simulink model "trajectory_test"  (R2021b)
settings: Solver=VariableStepAuto  StartTime=0.0  StopTime=65  RelTol=1e-3
settings Model: Creator=brian  LastModifiedBy=brian

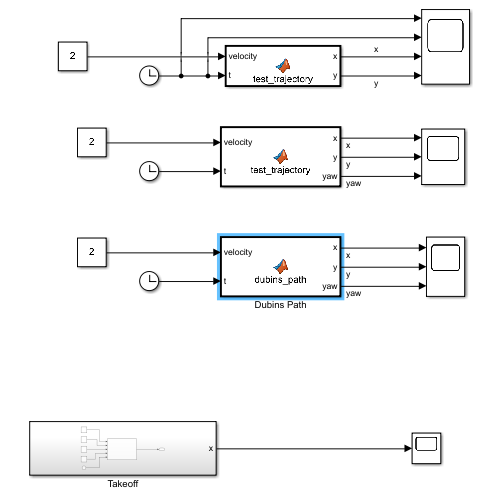
[thumbnail: Simulink's stored preview of the top-level diagram]
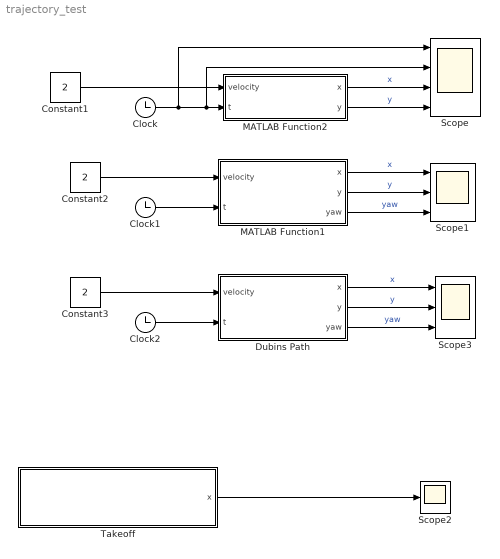
== system trajectory_test ==
  Clock : Clock
  Clock1 : Clock
  Clock2 : Clock
  Constant1 : Constant  Value=2
  Constant2 : Constant  Value=2
  Constant3 : Constant  Value=2
  Dubins Path : MATLAB Function  TreatAsAtomicUnit=on  SystemSampleTime=0.001
  MATLAB Function1 : MATLAB Function  TreatAsAtomicUnit=on  SystemSampleTime=0.001
  MATLAB Function2 : MATLAB Function  TreatAsAtomicUnit=on
  Scope : Scope  NumInputPorts=4
  Scope1 : Scope  NumInputPorts=3
  Scope2 : Scope
  Scope3 : Scope  NumInputPorts=3
  Takeoff : Subsystem
  wires:
  MATLAB Function2/2(y) -> Scope/4  "y"
  MATLAB Function2/1(x) -> Scope/3  "x"
  Clock/1 -> Scope/1, MATLAB Function2/2(t), Scope/2
  Constant1/1 -> MATLAB Function2/1(velocity)
  Takeoff/1(x) -> Scope2/1
  MATLAB Function1/3(yaw) -> Scope1/3  "yaw"
  MATLAB Function1/1(x) -> Scope1/1  "x"
  Clock1/1 -> MATLAB Function1/2(t)
  Constant2/1 -> MATLAB Function1/1(velocity)
  MATLAB Function1/2(y) -> Scope1/2  "y"
  Constant3/1 -> Dubins Path/1(velocity)
  Dubins Path/2(y) -> Scope3/2  "y"
  Dubins Path/3(yaw) -> Scope3/3  "yaw"
  Clock2/1 -> Dubins Path/2(t)
  Dubins Path/1(x) -> Scope3/1  "x"

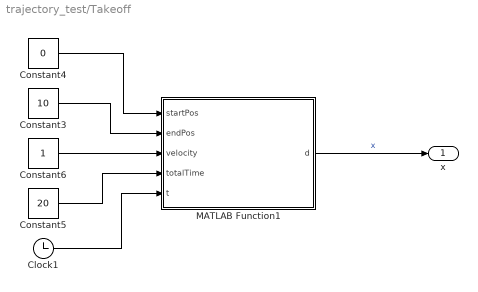
== system trajectory_test/Takeoff ==
  Clock1 : Clock
  Constant3 : Constant  Value=10
  Constant4 : Constant  Value=0
  Constant5 : Constant  Value=20
  Constant6 : Constant
  MATLAB Function1 : MATLAB Function  TreatAsAtomicUnit=on
  x : Outport
  wires:
  Constant3/1 -> MATLAB Function1/2(endPos)
  Constant6/1 -> MATLAB Function1/3(velocity)
  MATLAB Function1/1(d) -> x/1  "x"
  Constant5/1 -> MATLAB Function1/4(totalTime)
  Clock1/1 -> MATLAB Function1/5(t)
  Constant4/1 -> MATLAB Function1/1(startPos)

== matlab function trajectory_test/MATLAB Function2 ==
  settings: updateMethod=DISCRETE
  data: velocity input; x output; t input; y output

function [x, y] = test_trajectory(velocity, t)
    x = LSPB(0, 72, t, velocity, 40);
    if (t < 40)
        y = 0;
    else
        yt = t - 40;
        y = LSPB(0, 110, yt, velocity, 60);
    end
end

== matlab function trajectory_test/MATLAB Function1 ==
  settings: updateMethod=DISCRETE
  data: velocity input; x output; t input; y output; yaw output

% function [x, y] = test_trajectory(velocity, t)
%     x = LSPB(0, 72, t, velocity*2, 20);
%     y = 0;
% end

function [x, y, yaw] = test_trajectory(velocity, t)
    x = LSPB(0, 76.4, t, velocity*2, 20);
    if (t < 32)
        y = 0;
    else
        yt = t - 32;
        y = LSPB(0, 108, yt, velocity*2, 30);
    end
    if (t<=25)
        yaw = 0;
    else
        yawt = t - 25;
        yaw = LSPB(0,pi/2,yawt,0.5,5.0);
    end
end

== matlab function trajectory_test/Takeoff/MATLAB Function1 ==
  settings: updateMethod=DISCRETE
  data: startPos input; endPos input; velocity input; totalTime input; d output; t input
function d = test_trajectory(startPos, endPos, velocity, totalTime, t)
d = LSPB(startPos, endPos, t, velocity, totalTime);
end

== matlab function trajectory_test/Dubins Path ==
  settings: updateMethod=DISCRETE
  data: velocity input; x output; t input; y output; yaw output


function [x, y, yaw] = dubins_path(velocity, t)
    persistent time_offset1 time_offset2 radius turn_time
    if isempty(time_offset2)
        time_offset1 = 20;
        time_offset2 = 24;
        radius = 24.0;
        turn_time = 10.0;
    end

    if (t < time_offset1)
        x = LSPB(0, 76.4, t, velocity*2, 20);
        y = 0;
        yaw = 0;
        if (x >= (76.4-radius))
            time_offset1 = t;
            time_offset2 = time_offset1 + turn_time;
        end
    elseif (t < time_offset2)
        theta = ((pi/2) / (time_offset2 - time_offset1)) * (t-time_offset1);
        x = radius*sin(theta) - radius + 76.4;
        y = radius - radius*cos(theta);
        yaw = theta;
    else
        yt = t-time_offset2+7.5;
        x = 76.4;
        y = LSPB(0, 108, yt, velocity*2, 30);
        yaw = pi/2;
    end
end
